simulink model "Sistema"  (R2023a)
settings: Solver=ode45  StartTime=0.0  StopTime=10  MaxStep=1E-3  RelTol=1e-3
settings Model: LastModifiedBy=diegt
settings DataIOCC: ReturnWorkspaceOutputs=off  TimeSaveName=t
settings DebuggingCC: AlgebraicLoopMsg=none  ArtificialAlgebraicLoopMsg=none  MaxConsecutiveZCsMsg=none  ModelReferenceExtraNoncontSigs=none  OperatingPointInterfaceChecksumMismatchMsg=none
settings RTWCC: GPUComputeCapability=5.0

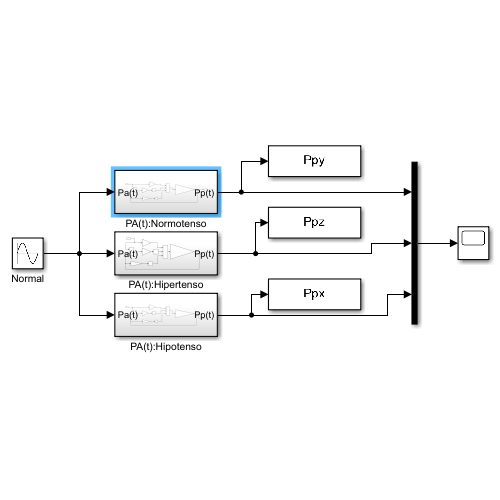
[thumbnail: Simulink's stored preview of the top-level diagram]
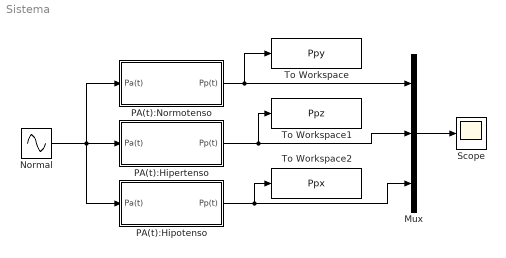
== system Sistema ==
  Mux : Mux  Inputs=3
  Normal : Sin  Bias=0.8  Frequency=((2*pi)*(95/60))
  PA(t):Hipertenso : Subsystem
  PA(t):Hipotenso : Subsystem
  PA(t):Normotenso : Subsystem
  Scope : Scope
  To Workspace : ToWorkspace  VariableName=Ppy  SampleTime=-1
  To Workspace1 : ToWorkspace  VariableName=Ppz  SampleTime=-1
  To Workspace2 : ToWorkspace  VariableName=Ppx  SampleTime=-1
  wires:
  Mux/1 -> Scope/1
  Normal/1 -> PA(t):Hipotenso/1(Pa(t)), PA(t):Hipertenso/1(Pa(t)), PA(t):Normotenso/1(Pa(t))
  PA(t):Normotenso/1(Pp(t)) -> Mux/1, To Workspace/1
  PA(t):Hipotenso/1(Pp(t)) -> To Workspace2/1, Mux/3
  PA(t):Hipertenso/1(Pp(t)) -> To Workspace1/1, Mux/2

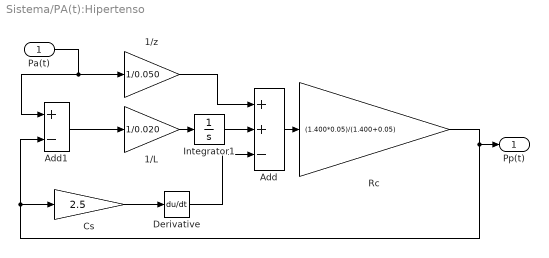
== system Sistema/PA(t):Hipertenso ==
  Pa(t) : Inport
  1/L : Gain  Gain=1/0.020
  1/z : Gain  Gain=1/0.050
  Add : Sum  Inputs=++-
  Add1 : Sum  Inputs=+-
  Cs : Gain  Gain=2.5
  Derivative : Derivative
  Integrator1 : Integrator
  Rc : Gain  Gain=(1.400*0.05)/(1.400+0.05)
  Pp(t) : Outport
  wires:
  Pa(t)/1 -> Add1/1, 1/z/1
  1/z/1 -> Add/1
  Add/1 -> Rc/1
  Add1/1 -> 1/L/1
  Rc/1 -> Pp(t)/1, Cs/1, Add1/2
  Cs/1 -> Derivative/1
  Integrator1/1 -> Add/2
  1/L/1 -> Integrator1/1
  Derivative/1 -> Add/3

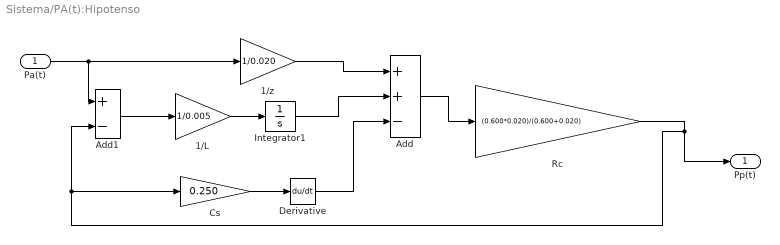
== system Sistema/PA(t):Hipotenso ==
  Pa(t) : Inport
  1/L : Gain  Gain=1/0.005
  1/z : Gain  Gain=1/0.020
  Add : Sum  Inputs=++-
  Add1 : Sum  Inputs=+-
  Cs : Gain  Gain=0.250
  Derivative : Derivative
  Integrator1 : Integrator
  Rc : Gain  Gain=(0.600*0.020)/(0.600+0.020)
  Pp(t) : Outport
  wires:
  Pa(t)/1 -> Add1/1, 1/z/1
  1/z/1 -> Add/1
  Add1/1 -> 1/L/1
  Rc/1 -> Cs/1, Add1/2, Pp(t)/1
  Cs/1 -> Derivative/1
  Integrator1/1 -> Add/2
  1/L/1 -> Integrator1/1
  Derivative/1 -> Add/3
  Add/1 -> Rc/1

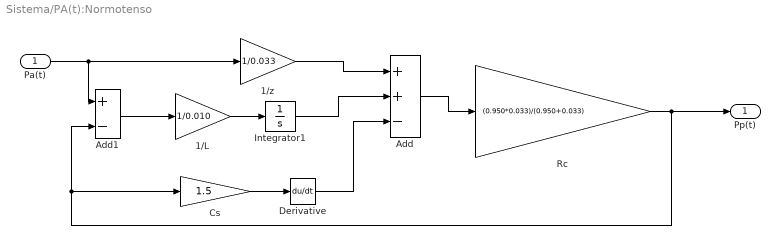
== system Sistema/PA(t):Normotenso ==
  Pa(t) : Inport
  1/L : Gain  Gain=1/0.010
  1/z : Gain  Gain=1/0.033
  Add : Sum  Inputs=++-
  Add1 : Sum  Inputs=+-
  Cs : Gain  Gain=1.5
  Derivative : Derivative
  Integrator1 : Integrator
  Rc : Gain  Gain=(0.950*0.033)/(0.950+0.033)
  Pp(t) : Outport
  wires:
  Pa(t)/1 -> Add1/1, 1/z/1
  1/z/1 -> Add/1
  Add/1 -> Rc/1
  Add1/1 -> 1/L/1
  Rc/1 -> Pp(t)/1, Cs/1, Add1/2
  Cs/1 -> Derivative/1
  Integrator1/1 -> Add/2
  1/L/1 -> Integrator1/1
  Derivative/1 -> Add/3
